simulink model "CubeSat_Archiv"  (R2019a)
settings: Solver=VariableStepAuto  StartTime=0.0  StopTime=10.0  RelTol=1e-3
undefined symbols (not defined in the file): D_distri, G_g, G_s, G_t, Gs, I_rw, I_vscmg, I_w, J_w, Kc, Ki, Kp, Kv, Kw_d, Kw_i, Kw_p, m, OMEGA_0, quat_0, smiData, tau_sat_mt, w_rw_ref, X, Y, Z
libraries: sm_lib x57, nesl_utility x28, aerolibutil x18, sharedtransform x5, ADCS_lib x4, simulink x2, sharedutil x2
(part 2 of 4)

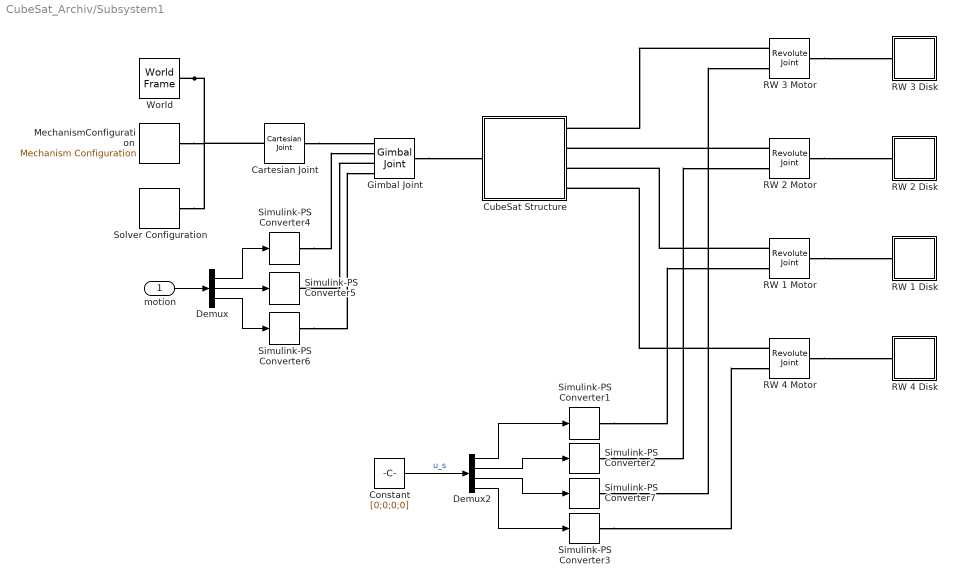
== system CubeSat_Archiv/Subsystem1 ==
  motion : Inport
  Cartesian Joint : sm_lib/Joints/Cartesian Joint  SenseConstraintForce=off  SenseConstraintForceX=off  SenseConstraintForceY=off  SenseConstraintForceZ=off  SenseConstraintTorque=off  SenseConstraintTorqueX=off  SenseConstraintTorqueY=off  SenseConstraintTorqueZ=off  SenseTotalForce=off  SenseTotalForceX=off  SenseTotalForceY=off  SenseTotalForceZ=off  SenseTotalTorque=off  SenseTotalTorqueX=off  SenseTotalTorqueY=off  SenseTotalTorqueZ=off  CompositeWrenchDir=FollowerOnBase  CompositeWrenchFrame=BaseFrame  PxEquilibriumPosition=0  PxEquilibriumPositionUnits=m  PxSpringStiffness=0  PxSpringStiffnessUnits=N/m  PxDampingCoefficient=0  PxDampingCoefficientUnits=N/(m/s)  PxTorqueActuationMode=NoTorque  PxMotionActuationMode=ComputedMotion  PxSensePosition=off  PxSenseVelocity=off  PxSenseAcceleration=off  PxSenseTorqueForce=off  PxSenseLowerLimitTorqueForce=off  PxSenseUpperLimitTorqueForce=off  PxLowerLimitSpecify=off  PxLowerLimitBound=-1  PxLowerLimitBoundUnits=m  PxLowerLimitStiffness=1e6  PxLowerLimitStiffnessUnits=N/m  PxLowerLimitDamping=1e3  PxLowerLimitDampingUnits=N/(m/s)  PxLowerLimitTransitionRegionWidth=1e-4  PxLowerLimitTransitionRegionWidthUnits=m  PxUpperLimitSpecify=off  PxUpperLimitBound=1  PxUpperLimitBoundUnits=m  PxUpperLimitStiffness=1e6  PxUpperLimitStiffnessUnits=N/m  PxUpperLimitDamping=1e3  PxUpperLimitDampingUnits=N/(m/s)  PxUpperLimitTransitionRegionWidth=1e-4  PxUpperLimitTransitionRegionWidthUnits=m  PxPositionTargetSpecify=off  PxPositionTargetPriority=High  PxPositionTargetValue=0  PxPositionTargetValueUnits=m  PxVelocityTargetSpecify=off  PxVelocityTargetPriority=High  PxVelocityTargetValue=0  PxVelocityTargetValueUnits=m/s  PyEquilibriumPosition=0  PyEquilibriumPositionUnits=m  PySpringStiffness=0  PySpringStiffnessUnits=N/m  PyDampingCoefficient=0  PyDampingCoefficientUnits=N/(m/s)  PyTorqueActuationMode=NoTorque  PyMotionActuationMode=ComputedMotion  PySensePosition=off  PySenseVelocity=off  PySenseAcceleration=off  PySenseTorqueForce=off  PySenseLowerLimitTorqueForce=off  PySenseUpperLimitTorqueForce=off  PyLowerLimitSpecify=off  PyLowerLimitBound=-1  PyLowerLimitBoundUnits=m  PyLowerLimitStiffness=1e6  PyLowerLimitStiffnessUnits=N/m  PyLowerLimitDamping=1e3  PyLowerLimitDampingUnits=N/(m/s)  PyLowerLimitTransitionRegionWidth=1e-4  PyLowerLimitTransitionRegionWidthUnits=m  PyUpperLimitSpecify=off  PyUpperLimitBound=1  PyUpperLimitBoundUnits=m  PyUpperLimitStiffness=1e6  PyUpperLimitStiffnessUnits=N/m  PyUpperLimitDamping=1e3  PyUpperLimitDampingUnits=N/(m/s)  PyUpperLimitTransitionRegionWidth=1e-4  PyUpperLimitTransitionRegionWidthUnits=m  PyPositionTargetSpecify=off  PyPositionTargetPriority=High  PyPositionTargetValue=0  PyPositionTargetValueUnits=m  PyVelocityTargetSpecify=off  PyVelocityTargetPriority=High  PyVelocityTargetValue=0  PyVelocityTargetValueUnits=m/s  PzEquilibriumPosition=0  PzEquilibriumPositionUnits=m  PzSpringStiffness=0  PzSpringStiffnessUnits=N/m  PzDampingCoefficient=0  PzDampingCoefficientUnits=N/(m/s)  PzTorqueActuationMode=NoTorque  PzMotionActuationMode=ComputedMotion  PzSensePosition=off  PzSenseVelocity=off  PzSenseAcceleration=off  PzSenseTorqueForce=off  PzSenseLowerLimitTorqueForce=off  PzSenseUpperLimitTorqueForce=off  PzLowerLimitSpecify=off  PzLowerLimitBound=-1  PzLowerLimitBoundUnits=m  PzLowerLimitStiffness=1e6  PzLowerLimitStiffnessUnits=N/m  PzLowerLimitDamping=1e3  PzLowerLimitDampingUnits=N/(m/s)  PzLowerLimitTransitionRegionWidth=1e-4  PzLowerLimitTransitionRegionWidthUnits=m  PzUpperLimitSpecify=off  PzUpperLimitBound=1  PzUpperLimitBoundUnits=m  PzUpperLimitStiffness=1e6  PzUpperLimitStiffnessUnits=N/m  PzUpperLimitDamping=1e3  PzUpperLimitDampingUnits=N/(m/s)  PzUpperLimitTransitionRegionWidth=1e-4  PzUpperLimitTransitionRegionWidthUnits=m  PzPositionTargetSpecify=off  PzPositionTargetPriority=High  PzPositionTargetValue=0  PzPositionTargetValueUnits=m  PzVelocityTargetSpecify=off  PzVelocityTargetPriority=High  PzVelocityTargetValue=0  PzVelocityTargetValueUnits=m/s
  Constant : Constant  Value=[0;0;0;0]
  CubeSat Structure : Subsystem
  Demux : Demux  Outputs=3
  Demux2 : Demux
  Gimbal Joint : sm_lib/Joints/Gimbal Joint  SenseConstraintForce=off  SenseConstraintForceX=off  SenseConstraintForceY=off  SenseConstraintForceZ=off  SenseConstraintTorque=off  SenseConstraintTorqueX=off  SenseConstraintTorqueY=off  SenseConstraintTorqueZ=off  SenseTotalForce=off  SenseTotalForceX=off  SenseTotalForceY=off  SenseTotalForceZ=off  SenseTotalTorque=off  SenseTotalTorqueX=off  SenseTotalTorqueY=off  SenseTotalTorqueZ=off  CompositeWrenchDir=FollowerOnBase  CompositeWrenchFrame=BaseFrame  RxEquilibriumPosition=0  RxEquilibriumPositionUnits=deg  RxSpringStiffness=0  RxSpringStiffnessUnits=N*m/deg  RxDampingCoefficient=0  RxDampingCoefficientUnits=N*m/(deg/s)  RxTorqueActuationMode=ComputedTorque  RxMotionActuationMode=InputMotion  RxSensePosition=off  RxSenseVelocity=off  RxSenseAcceleration=off  RxSenseTorqueForce=off  RxSenseLowerLimitTorqueForce=off  RxSenseUpperLimitTorqueForce=off  RxLowerLimitSpecify=off  RxLowerLimitBound=-90  RxLowerLimitBoundUnits=deg  RxLowerLimitStiffness=1e4  RxLowerLimitStiffnessUnits=N*m/deg  RxLowerLimitDamping=10  RxLowerLimitDampingUnits=N*m/(deg/s)  RxLowerLimitTransitionRegionWidth=0.1  RxLowerLimitTransitionRegionWidthUnits=deg  RxUpperLimitSpecify=off  RxUpperLimitBound=90  RxUpperLimitBoundUnits=deg  RxUpperLimitStiffness=1e4  RxUpperLimitStiffnessUnits=N*m/deg  RxUpperLimitDamping=10  RxUpperLimitDampingUnits=N*m/(deg/s)  RxUpperLimitTransitionRegionWidth=0.1  RxUpperLimitTransitionRegionWidthUnits=deg  RxPositionTargetSpecify=off  RxPositionTargetPriority=High  RxPositionTargetValue=0  RxPositionTargetValueUnits=rad  RxVelocityTargetSpecify=off  RxVelocityTargetPriority=High  RxVelocityTargetValue=0  RxVelocityTargetValueUnits=deg/s  RyEquilibriumPosition=0  RyEquilibriumPositionUnits=deg  RySpringStiffness=0  RySpringStiffnessUnits=N*m/deg  RyDampingCoefficient=0  RyDampingCoefficientUnits=N*m/(deg/s)  RyTorqueActuationMode=ComputedTorque  RyMotionActuationMode=InputMotion  RySensePosition=off  RySenseVelocity=off  RySenseAcceleration=off  RySenseTorqueForce=off  RySenseLowerLimitTorqueForce=off  RySenseUpperLimitTorqueForce=off  RyLowerLimitSpecify=off  RyLowerLimitBound=-90  RyLowerLimitBoundUnits=deg  RyLowerLimitStiffness=1e4  RyLowerLimitStiffnessUnits=N*m/deg  RyLowerLimitDamping=10  RyLowerLimitDampingUnits=N*m/(deg/s)  RyLowerLimitTransitionRegionWidth=0.1  RyLowerLimitTransitionRegionWidthUnits=deg  RyUpperLimitSpecify=off  RyUpperLimitBound=90  RyUpperLimitBoundUnits=deg  RyUpperLimitStiffness=1e4  RyUpperLimitStiffnessUnits=N*m/deg  RyUpperLimitDamping=10  RyUpperLimitDampingUnits=N*m/(deg/s)  RyUpperLimitTransitionRegionWidth=0.1  RyUpperLimitTransitionRegionWidthUnits=deg  RyPositionTargetSpecify=off  RyPositionTargetPriority=High  RyPositionTargetValue=0  RyPositionTargetValueUnits=deg  RyVelocityTargetSpecify=off  RyVelocityTargetPriority=High  RyVelocityTargetValue=0  RyVelocityTargetValueUnits=deg/s  RzEquilibriumPosition=0  RzEquilibriumPositionUnits=deg  RzSpringStiffness=0  RzSpringStiffnessUnits=N*m/deg  RzDampingCoefficient=0  RzDampingCoefficientUnits=N*m/(deg/s)  RzTorqueActuationMode=ComputedTorque  RzMotionActuationMode=InputMotion  RzSensePosition=off  RzSenseVelocity=off  RzSenseAcceleration=off  RzSenseTorqueForce=off  RzSenseLowerLimitTorqueForce=off  RzSenseUpperLimitTorqueForce=off  RzLowerLimitSpecify=off  RzLowerLimitBound=-90  RzLowerLimitBoundUnits=deg  RzLowerLimitStiffness=1e4  RzLowerLimitStiffnessUnits=N*m/deg  RzLowerLimitDamping=10  RzLowerLimitDampingUnits=N*m/(deg/s)  RzLowerLimitTransitionRegionWidth=0.1  RzLowerLimitTransitionRegionWidthUnits=deg  RzUpperLimitSpecify=off  RzUpperLimitBound=90  RzUpperLimitBoundUnits=deg  RzUpperLimitStiffness=1e4  RzUpperLimitStiffnessUnits=N*m/deg  RzUpperLimitDamping=10  RzUpperLimitDampingUnits=N*m/(deg/s)  RzUpperLimitTransitionRegionWidth=0.1  RzUpperLimitTransitionRegionWidthUnits=deg  RzPositionTargetSpecify=off  RzPositionTargetPriority=High  RzPositionTargetValue=0  RzPositionTargetValueUnits=deg  RzVelocityTargetSpecify=off  RzVelocityTargetPriority=High  RzVelocityTargetValue=0  RzVelocityTargetValueUnits=deg/s
      settings: SourceProductName=Simscape Multibody
  MechanismConfiguration : sm_lib/Utilities/Mechanism Configuration  UniformGravity=None  GravityVector=[0 -9.80665 0]  GravityUnits=m/s^2  LinearizationDelta=0.001
  RW 1 Disk : Subsystem
  RW 1 Motor : sm_lib/Joints/Revolute Joint  SenseConstraintForce=off  SenseConstraintForceX=off  SenseConstraintForceY=off  SenseConstraintForceZ=off  SenseConstraintTorque=off  SenseConstraintTorqueX=off  SenseConstraintTorqueY=off  SenseConstraintTorqueZ=off  SenseTotalForce=off  SenseTotalForceX=off  SenseTotalForceY=off  SenseTotalForceZ=off  SenseTotalTorque=off  SenseTotalTorqueX=off  SenseTotalTorqueY=off  SenseTotalTorqueZ=off  CompositeWrenchDir=FollowerOnBase  CompositeWrenchFrame=BaseFrame  EquilibriumPosition=0  EquilibriumPositionUnits=rad  SpringStiffness=0  SpringStiffnessUnits=N*m/rad  DampingCoefficient=0  DampingCoefficientUnits=N*m/(rad/s)  TorqueActuationMode=InputTorque  MotionActuationMode=ComputedMotion  SensePosition=off  SenseVelocity=off  SenseAcceleration=off  SenseTorqueForce=off  SenseLowerLimitTorqueForce=off  SenseUpperLimitTorqueForce=off  LowerLimitSpecify=off  LowerLimitBound=-90  LowerLimitBoundUnits=deg  LowerLimitStiffness=1e4  LowerLimitStiffnessUnits=N*m/deg  LowerLimitDamping=10  LowerLimitDampingUnits=N*m/(deg/s)  LowerLimitTransitionRegionWidth=0.1  LowerLimitTransitionRegionWidthUnits=deg  UpperLimitSpecify=off  UpperLimitBound=90  UpperLimitBoundUnits=deg  UpperLimitStiffness=1e4  UpperLimitStiffnessUnits=N*m/deg  UpperLimitDamping=10  UpperLimitDampingUnits=N*m/(deg/s)  UpperLimitTransitionRegionWidth=0.1  UpperLimitTransitionRegionWidthUnits=deg  PositionTargetSpecify=off  PositionTargetPriority=Low  PositionTargetValue=smiData.RevoluteJoint(2).Rz.Pos  PositionTargetValueUnits=deg  VelocityTargetSpecify=off  VelocityTargetPriority=High  VelocityTargetValue=0  VelocityTargetValueUnits=deg/s
  RW 2 Disk : Subsystem
  RW 2 Motor : sm_lib/Joints/Revolute Joint  SenseConstraintForce=off  SenseConstraintForceX=off  SenseConstraintForceY=off  SenseConstraintForceZ=off  SenseConstraintTorque=off  SenseConstraintTorqueX=off  SenseConstraintTorqueY=off  SenseConstraintTorqueZ=off  SenseTotalForce=off  SenseTotalForceX=off  SenseTotalForceY=off  SenseTotalForceZ=off  SenseTotalTorque=off  SenseTotalTorqueX=off  SenseTotalTorqueY=off  SenseTotalTorqueZ=off  CompositeWrenchDir=FollowerOnBase  CompositeWrenchFrame=BaseFrame  EquilibriumPosition=0  EquilibriumPositionUnits=rad  SpringStiffness=0  SpringStiffnessUnits=N*m/rad  DampingCoefficient=0  DampingCoefficientUnits=N*m/(rad/s)  TorqueActuationMode=InputTorque  MotionActuationMode=ComputedMotion  SensePosition=off  SenseVelocity=off  SenseAcceleration=off  SenseTorqueForce=off  SenseLowerLimitTorqueForce=off  SenseUpperLimitTorqueForce=off  LowerLimitSpecify=off  LowerLimitBound=-90  LowerLimitBoundUnits=deg  LowerLimitStiffness=1e4  LowerLimitStiffnessUnits=N*m/deg  LowerLimitDamping=10  LowerLimitDampingUnits=N*m/(deg/s)  LowerLimitTransitionRegionWidth=0.1  LowerLimitTransitionRegionWidthUnits=deg  UpperLimitSpecify=off  UpperLimitBound=90  UpperLimitBoundUnits=deg  UpperLimitStiffness=1e4  UpperLimitStiffnessUnits=N*m/deg  UpperLimitDamping=10  UpperLimitDampingUnits=N*m/(deg/s)  UpperLimitTransitionRegionWidth=0.1  UpperLimitTransitionRegionWidthUnits=deg  PositionTargetSpecify=off  PositionTargetPriority=Low  PositionTargetValue=smiData.RevoluteJoint(3).Rz.Pos  PositionTargetValueUnits=deg  VelocityTargetSpecify=off  VelocityTargetPriority=High  VelocityTargetValue=0  VelocityTargetValueUnits=deg/s
  RW 3 Disk : Subsystem
  RW 3 Motor : sm_lib/Joints/Revolute Joint  SenseConstraintForce=off  SenseConstraintForceX=off  SenseConstraintForceY=off  SenseConstraintForceZ=off  SenseConstraintTorque=off  SenseConstraintTorqueX=off  SenseConstraintTorqueY=off  SenseConstraintTorqueZ=off  SenseTotalForce=off  SenseTotalForceX=off  SenseTotalForceY=off  SenseTotalForceZ=off  SenseTotalTorque=off  SenseTotalTorqueX=off  SenseTotalTorqueY=off  SenseTotalTorqueZ=off  CompositeWrenchDir=FollowerOnBase  CompositeWrenchFrame=BaseFrame  EquilibriumPosition=0  EquilibriumPositionUnits=rad  SpringStiffness=0  SpringStiffnessUnits=N*m/rad  DampingCoefficient=0  DampingCoefficientUnits=N*m/(rad/s)  TorqueActuationMode=InputTorque  MotionActuationMode=ComputedMotion  SensePosition=off  SenseVelocity=off  SenseAcceleration=off  SenseTorqueForce=off  SenseLowerLimitTorqueForce=off  SenseUpperLimitTorqueForce=off  LowerLimitSpecify=off  LowerLimitBound=-90  LowerLimitBoundUnits=deg  LowerLimitStiffness=1e4  LowerLimitStiffnessUnits=N*m/deg  LowerLimitDamping=10  LowerLimitDampingUnits=N*m/(deg/s)  LowerLimitTransitionRegionWidth=0.1  LowerLimitTransitionRegionWidthUnits=deg  UpperLimitSpecify=off  UpperLimitBound=90  UpperLimitBoundUnits=deg  UpperLimitStiffness=1e4  UpperLimitStiffnessUnits=N*m/deg  UpperLimitDamping=10  UpperLimitDampingUnits=N*m/(deg/s)  UpperLimitTransitionRegionWidth=0.1  UpperLimitTransitionRegionWidthUnits=deg  PositionTargetSpecify=off  PositionTargetPriority=Low  PositionTargetValue=smiData.RevoluteJoint(4).Rz.Pos  PositionTargetValueUnits=deg  VelocityTargetSpecify=off  VelocityTargetPriority=High  VelocityTargetValue=0  VelocityTargetValueUnits=deg/s
  RW 4 Disk : Subsystem
  RW 4 Motor : sm_lib/Joints/Revolute Joint  SenseConstraintForce=off  SenseConstraintForceX=off  SenseConstraintForceY=off  SenseConstraintForceZ=off  SenseConstraintTorque=off  SenseConstraintTorqueX=off  SenseConstraintTorqueY=off  SenseConstraintTorqueZ=off  SenseTotalForce=off  SenseTotalForceX=off  SenseTotalForceY=off  SenseTotalForceZ=off  SenseTotalTorque=off  SenseTotalTorqueX=off  SenseTotalTorqueY=off  SenseTotalTorqueZ=off  CompositeWrenchDir=FollowerOnBase  CompositeWrenchFrame=BaseFrame  EquilibriumPosition=0  EquilibriumPositionUnits=rad  SpringStiffness=0  SpringStiffnessUnits=N*m/rad  DampingCoefficient=0  DampingCoefficientUnits=N*m/(rad/s)  TorqueActuationMode=InputTorque  MotionActuationMode=ComputedMotion  SensePosition=off  SenseVelocity=off  SenseAcceleration=off  SenseTorqueForce=off  SenseLowerLimitTorqueForce=off  SenseUpperLimitTorqueForce=off  LowerLimitSpecify=off  LowerLimitBound=-90  LowerLimitBoundUnits=deg  LowerLimitStiffness=1e4  LowerLimitStiffnessUnits=N*m/deg  LowerLimitDamping=10  LowerLimitDampingUnits=N*m/(deg/s)  LowerLimitTransitionRegionWidth=0.1  LowerLimitTransitionRegionWidthUnits=deg  UpperLimitSpecify=off  UpperLimitBound=90  UpperLimitBoundUnits=deg  UpperLimitStiffness=1e4  UpperLimitStiffnessUnits=N*m/deg  UpperLimitDamping=10  UpperLimitDampingUnits=N*m/(deg/s)  UpperLimitTransitionRegionWidth=0.1  UpperLimitTransitionRegionWidthUnits=deg  PositionTargetSpecify=off  PositionTargetPriority=Low  PositionTargetValue=smiData.RevoluteJoint(1).Rz.Pos  PositionTargetValueUnits=deg  VelocityTargetSpecify=off  VelocityTargetPriority=High  VelocityTargetValue=0  VelocityTargetValueUnits=deg/s
  Simulink-PS Converter{1,4..6} (4 alike) : nesl_utility/Simulink-PS Converter  PhysicalDomain=network_engine_domain  SubClassName=ps_input  LeftPortType=input  RightPortType=output  PseudoPeriodic=off  Frequencies=[]  NoiseDistribution=none  NoiseParameters=[]  Unit=1  AffineConversion=off  FilteringAndDerivatives=filter  SimscapeFilterOrder=2  InputFilterTimeConstant=0.001  UdotUserProvided=1
  Simulink-PS Converter2 : nesl_utility/Simulink-PS Converter  PhysicalDomain=network_engine_domain  SubClassName=ps_input  LeftPortType=input  RightPortType=output  PseudoPeriodic=off  Frequencies=[]  NoiseDistribution=none  NoiseParameters=[]  Unit=1  AffineConversion=off  FilteringAndDerivatives=filter  SimscapeFilterOrder=2  InputFilterTimeConstant=0.001  UdotUserProvided=0
  Simulink-PS Converter3 : nesl_utility/Simulink-PS Converter  PhysicalDomain=network_engine_domain  SubClassName=ps_input  LeftPortType=input  RightPortType=output  PseudoPeriodic=off  Frequencies=[]  NoiseDistribution=none  NoiseParameters=[]  Unit=1  AffineConversion=off  FilteringAndDerivatives=filter  SimscapeFilterOrder=2  InputFilterTimeConstant=0.001  UdotUserProvided=0
  Simulink-PS Converter7 : nesl_utility/Simulink-PS Converter  PhysicalDomain=network_engine_domain  SubClassName=ps_input  LeftPortType=input  RightPortType=output  PseudoPeriodic=off  Frequencies=[]  NoiseDistribution=none  NoiseParameters=[]  Unit=1  AffineConversion=off  FilteringAndDerivatives=filter  SimscapeFilterOrder=2  InputFilterTimeConstant=0.001  UdotUserProvided=0
  Solver Configuration : nesl_utility/Solver Configuration  PhysicalDomain=network_engine_domain  SubClassName=solver  LeftPortType=input  RightPortType=generic  Tones=[]  Harmonics=[]  SimulateNoise=off  Profile=off  UseLocalSampling=off  EnableSwitchedLinearOptims=on  FrequencyDomain=off  UseCCode=off  RelTol=0.001  AbsTol=1e-06  MinStep=1e-09  ToWorkspace=off  RevertToSquareIcSolve=off  NumHomotopyIterations=100  PhasorMode=off  PhasorModeNumHarmonics=1  DoDC=off  ResidualTolerance=1e-09  UseLocalSolver=off  LocalSolverChoice=NE_BACKWARD_EULER_ADVANCER  LocalSolverSampleTime=0.001  DoFixedCost=off  MaxNonlinIter=3  MaxModeIter=2  LinearAlgebra=Sparse  EquationFormulation=NE_TIME_EF  DelaysMemoryBudget=1024  AutomaticFiltering=on  FilteringTimeConstant=0.001  PartitionStorageMethod=AS_NEEDED  PartitionMemoryBudget=1024  PartitionMethod=FAST
  World : sm_lib/Frames and Transforms/World Frame
  wires:
  Demux2/2 -> Simulink-PS Converter2/1
  Demux2/3 -> Simulink-PS Converter7/1
  Demux2/4 -> Simulink-PS Converter3/1
  Demux2/1 -> Simulink-PS Converter1/1
  Constant/1 -> Demux2/1  "u_s"
  Demux/2 -> Simulink-PS Converter5/1
  Demux/1 -> Simulink-PS Converter4/1
  Demux/3 -> Simulink-PS Converter6/1
  motion/1 -> Demux/1
  connections:
  World/RConn1 -- Cartesian Joint/LConn1 -- Solver Configuration/RConn1 -- MechanismConfiguration/RConn1
  Simulink-PS Converter3/RConn1 -- RW 4 Motor/LConn2
  RW 3 Motor/RConn1 -- RW 3 Disk/LConn1
  Simulink-PS Converter1/RConn1 -- RW 1 Motor/LConn2
  Simulink-PS Converter7/RConn1 -- RW 3 Motor/LConn2
  RW 2 Motor/RConn1 -- RW 2 Disk/LConn1
  Simulink-PS Converter2/RConn1 -- RW 2 Motor/LConn2
  RW 1 Motor/RConn1 -- RW 1 Disk/LConn1
  RW 4 Motor/LConn1 -- CubeSat Structure/RConn4
  RW 1 Motor/LConn1 -- CubeSat Structure/RConn3
  RW 3 Motor/LConn1 -- CubeSat Structure/RConn1
  RW 4 Motor/RConn1 -- RW 4 Disk/LConn1
  RW 2 Motor/LConn1 -- CubeSat Structure/RConn2
  Gimbal Joint/RConn1 -- CubeSat Structure/LConn1
  Cartesian Joint/RConn1 -- Gimbal Joint/LConn1
  Simulink-PS Converter4/RConn1 -- Gimbal Joint/LConn2
  Gimbal Joint/LConn3 -- Simulink-PS Converter5/RConn1
  Simulink-PS Converter6/RConn1 -- Gimbal Joint/LConn4

== system CubeSat_Archiv/vscmg dynamics v1.0 ==
  note: VSCMG Eqn
  In1 : Inport
  In2 : Inport  Port=2
  Dynamics VSCMG : Subsystem
  Kinematics1 : Subsystem
  OMEGA_vscmg : Scope
  VSCMGC : Subsystem
  omega_w_vscmg : Scope
  Out1 : Outport
  wires:
  Kinematics1/1(q) -> Out1/1
  In2/1 -> Dynamics VSCMG/3(ext.torq)
  Dynamics VSCMG/1(OMEGA) -> OMEGA_vscmg/1, Kinematics1/1(OMEGA)
  Dynamics VSCMG/2(ALPHA) -> VSCMGC/1(ALPHA)
  VSCMGC/2(alpha_w) -> Dynamics VSCMG/2(alpha_w)
  In1/1 -> VSCMGC/2(tau_cmd)
  VSCMGC/1(omega_w) -> Dynamics VSCMG/1(omega_w), omega_w_vscmg/1

== system CubeSat_Archiv/Actuator/Magnetic Torquer Cluster ==
  b_t_cmd_mtc : Inport
  Envi : Inport  Port=2
  Terminator : Terminator
  Out1 : Outport
  wires:
  b_t_cmd_mtc/1 -> Out1/1
  Envi/1 -> Terminator/1

== system CubeSat_Archiv/Actuator/Reaction Wheel Cluster ==
  b_w_b/n : Inport
  b_a_b/n : Inport  Port=2
  b_t_cmd_rwc : Inport  Port=3
  Demux : Demux
  Distri Mtx2 : Gain  Gain=D_distri  Multiplication=Matrix(K*u)
  Mux1 : Mux
  Mux2 : Mux
  RW 1 : Subsystem
  RW 2 : Subsystem
  RW 3 : Subsystem
  RW 4 : Subsystem
  h_s : Outport
  u_s : Outport  Port=2
  omega_w : Outport  Port=3
  wires:
  Demux/3 -> RW 3/3(u_s_3)
  Demux/1 -> RW 1/3(u_s_1)
  Demux/2 -> RW 2/3(u_s_2)
  Demux/4 -> RW 4/3(u_s_4)
  b_t_cmd_rwc/1 -> Distri Mtx2/1
  b_a_b/n/1 -> RW 4/2(ALPHA), RW 3/2(ALPHA), RW 2/2(ALPHA), RW 1/2(ALPHA)
  RW 1/2(omega_w_1) -> Mux2/1
  Distri Mtx2/1 -> u_s/1, Demux/1  "u_s"
  RW 4/1(h_w_4) -> Mux1/4
  RW 1/1(h_w_1) -> Mux1/1
  Mux2/1 -> omega_w/1
  Mux1/1 -> h_s/1
  RW 3/2(omega_w_3) -> Mux2/3
  RW 4/2(omega_w_4) -> Mux2/4
  b_w_b/n/1 -> RW 4/1(OMEGA), RW 3/1(OMEGA), RW 2/1(OMEGA), RW 1/1(OMEGA)
  RW 3/1(h_w_3) -> Mux1/3
  RW 2/2(omega_w_2) -> Mux2/2
  RW 2/1(h_w_2) -> Mux1/2

== system CubeSat_Archiv/Controller1/LQI_Full State_Verified1 ==
  In Bus Element2 : Inport  PortName=RefState  Element=q_eci2r
  In Bus Element : Inport  Port=2  PortName=SensorIn  Element=q_eci2b
  In Bus Element7 : Inport  Port=2  PortName=SensorIn  Element=b_w_b/n
  Add2 : Sum  Inputs=|+-
  Atti Err : Subsystem  AncestorBlock=ADCS_lib/PIV/Atti Err
  Integrator1 : Integrator
  Kc Ctrl Gain : Gain  Gain=-Kc  Multiplication=Matrix(K*u)
  Ki Integral Gain : Gain  Gain=Ki  Multiplication=Matrix(K*u)
  Vector Concatenate : Concatenate
  Vector Concatenate1 : Concatenate
  Vector Out Unwinding1 : Subsystem
  vector part1 : Selector  InputPortWidth=4  IndexOptions=Index vector (dialog)  Indices=[2 3 4]  OutputSizes=1
  CtrlCmd : Outport
  Out Bus Element : Outport  Port=2  PortName=CtrlState  Element=q_r2b
  wires:
  Ki Integral Gain/1 -> Add2/1
  Atti Err/1(q_r2b) -> Out Bus Element/1, Vector Out Unwinding1/1(q)
  In Bus Element/1 -> vector part1/1, Atti Err/2(q_eci2b)
  In Bus Element2/1 -> Atti Err/1(q_eci2r)
  Kc Ctrl Gain/1 -> Add2/2
  Add2/1 -> CtrlCmd/1
  Integrator1/1 -> Ki Integral Gain/1
  vector part1/1 -> Vector Concatenate/1
  Vector Concatenate/1 -> Kc Ctrl Gain/1
  In Bus Element7/1 -> Vector Concatenate/2, Vector Concatenate1/2
  Vector Out Unwinding1/1(ε) -> Vector Concatenate1/1
  Vector Concatenate1/1 -> Integrator1/1

== system CubeSat_Archiv/Controller1/Momentum Management ==
  CtrlCmd : Inport
  w_rw : Inport  Port=2
  Add : Sum  Inputs=|++
  G_s : Gain  Gain=G_s  Multiplication=Matrix(K*u)
  de-spin torq : Subsystem
  b_t_cmd_rwc : Outport
  b_t_cmd_mtc : Outport  Port=2
  wires:
  de-spin torq/1(u_despin) -> G_s/1
  w_rw/1 -> de-spin torq/1(w_rw)
  Add/1 -> b_t_cmd_rwc/1
  G_s/1 -> b_t_cmd_mtc/1, Add/2
  CtrlCmd/1 -> Add/1

== system CubeSat_Archiv/Dynamics/integrate quaternion ==
  b_w_b/n : Inport
  Constant : Constant  Value=0
  Gain : Gain  Gain=0.5
  Integrator : Integrator  InitialCondition=quat_0
  Quaternion Multiplication : aerolibutil/Quaternion Multiplication
  Vector Concatenate : Concatenate
  q_eci2b : Outport
  wires:
  Quaternion Multiplication/1 -> Integrator/1
  b_w_b/n/1 -> Vector Concatenate/2
  Integrator/1 -> q_eci2b/1, Gain/1
  Gain/1 -> Quaternion Multiplication/1
  Vector Concatenate/1 -> Quaternion Multiplication/2
  Constant/1 -> Vector Concatenate/1

== system CubeSat_Archiv/Dynamics without FF/Integrate Quaternion KDE ==
  b_w_b/n : Inport
  Constant : Constant  Value=0
  Gain : Gain  Gain=0.5
  Integrator : Integrator  InitialCondition=quat_0
  Quaternion Multiplication : aerolibutil/Quaternion Multiplication
  Quaternion Normalize : sharedutil/Quaternion Normalize  aMode=aMode
      settings: SourceProductName=Aerospace Blockset  SourceProductBaseCode=AE
  Vector Concatenate : Concatenate
  q_eci2b : Outport
  wires:
  Quaternion Normalize/1 -> q_eci2b/1
  Constant/1 -> Vector Concatenate/1
  Vector Concatenate/1 -> Quaternion Multiplication/2
  Gain/1 -> Quaternion Multiplication/1
  Integrator/1 -> Gain/1, Quaternion Normalize/1
  b_w_b/n/1 -> Vector Concatenate/2
  Quaternion Multiplication/1 -> Integrator/1

== system CubeSat_Archiv/FeedFwd/RW 1 ==
  OMEGA : Inport
  omega_w_1 : Inport  Port=2
  Gain2 : Gain  Gain=G_s(:,1).'  Multiplication=Matrix(K*u)
  I_w : Gain  Gain=I_w(1,1)
  Sum1 : Sum
  h_w_1 : Outport
  wires:
  omega_w_1/1 -> Sum1/2
  Sum1/1 -> I_w/1
  I_w/1 -> h_w_1/1
  Gain2/1 -> Sum1/1
  OMEGA/1 -> Gain2/1

== system CubeSat_Archiv/FeedFwd/RW 2 ==
  OMEGA : Inport
  omega_w_1 : Inport  Port=2
  Gain2 : Gain  Gain=G_s(:,1).'  Multiplication=Matrix(K*u)
  I_w : Gain  Gain=I_w(1,1)
  Sum1 : Sum
  h_w_1 : Outport
  wires:
  OMEGA/1 -> Gain2/1
  Gain2/1 -> Sum1/1
  I_w/1 -> h_w_1/1
  Sum1/1 -> I_w/1
  omega_w_1/1 -> Sum1/2

== system CubeSat_Archiv/FeedFwd/RW 3 ==
  OMEGA : Inport
  omega_w_1 : Inport  Port=2
  Gain2 : Gain  Gain=G_s(:,1).'  Multiplication=Matrix(K*u)
  I_w : Gain  Gain=I_w(1,1)
  Sum1 : Sum
  h_w_1 : Outport
  wires:
  omega_w_1/1 -> Sum1/2
  Sum1/1 -> I_w/1
  I_w/1 -> h_w_1/1
  Gain2/1 -> Sum1/1
  OMEGA/1 -> Gain2/1

== system CubeSat_Archiv/FeedFwd/RW 4 ==
  OMEGA : Inport
  omega_w_1 : Inport  Port=2
  Gain2 : Gain  Gain=G_s(:,1).'  Multiplication=Matrix(K*u)
  I_w : Gain  Gain=I_w(1,1)
  Sum1 : Sum
  h_w_1 : Outport
  wires:
  OMEGA/1 -> Gain2/1
  Gain2/1 -> Sum1/1
  I_w/1 -> h_w_1/1
  Sum1/1 -> I_w/1
  omega_w_1/1 -> Sum1/2

== system CubeSat_Archiv/LQI_Full State_Verified/Atti Err1 ==
  q_eci2r : Inport
  q_eci2b : Inport  Port=2
  Quaternion Inverse1 : aerolibutil/Quaternion Inverse
      settings: SourceProductName=Aerospace Blockset
  Quaternion Multiplication : aerolibutil/Quaternion Multiplication
  "[BR]" : sharedtransform/Quaternions to  Direction Cosine Matrix  aMode=aMode
      settings: SourceProductName=Aerospace Blockset  SourceProductBaseCode=AE
  q_r2b : Outport
  DCM : Outport  Port=2
  wires:
  Quaternion Inverse1/1 -> Quaternion Multiplication/1
  "[BR]"/1 -> DCM/1
  q_eci2r/1 -> Quaternion Multiplication/2
  q_eci2b/1 -> Quaternion Inverse1/1
  Quaternion Multiplication/1 -> "[BR]"/1, q_r2b/1

== system CubeSat_Archiv/LQI_Full State_Verified/Vector Out Unwinding1 ==
  q : Inport
  Product2 : Product
  Short Rotation : Subsystem
  vector part : Selector  InputPortWidth=4  IndexOptions=Index vector (dialog)  Indices=[2 3 4]  OutputSizes=1
  ε : Outport
  wires:
  Product2/1 -> ε/1
  Short Rotation/1(sgn) -> Product2/1
  q/1 -> Short Rotation/1(q), vector part/1
  vector part/1 -> Product2/2

== system CubeSat_Archiv/LQI_Full State_Verified/r2b ==
  "[BR]" : Inport
  r_w_r/n : Inport  Port=2
  Derivative : Derivative
  Product : Product  Multiplication=Matrix(*)
  Product1 : Product  Multiplication=Matrix(*)
  b_w_r/n : Outport
  b_a_r/n : Outport  Port=2
  wires:
  Product/1 -> b_w_r/n/1
  Product1/1 -> b_a_r/n/1
  Derivative/1 -> Product1/2  "r_a_r/n"
  "[BR]"/1 -> Product/1, Product1/1
  r_w_r/n/1 -> Derivative/1, Product/2

== system CubeSat_Archiv/LQI_Half State_Don't Use!/Atti Err1 ==
  q_eci2r : Inport
  q_eci2b : Inport  Port=2
  Quaternion Inverse1 : aerolibutil/Quaternion Inverse
      settings: SourceProductName=Aerospace Blockset
  Quaternion Multiplication : aerolibutil/Quaternion Multiplication
  q_r2b : Outport
  wires:
  Quaternion Multiplication/1 -> q_r2b/1
  q_eci2b/1 -> Quaternion Inverse1/1
  q_eci2r/1 -> Quaternion Multiplication/2
  Quaternion Inverse1/1 -> Quaternion Multiplication/1

== system CubeSat_Archiv/LQI_Half State_Don't Use!/Vector Out Unwinding2 ==
  q : Inport
  Product2 : Product
  Short Rotation : Subsystem
  vector part : Selector  InputPortWidth=4  IndexOptions=Index vector (dialog)  Indices=[2 3 4]  OutputSizes=1
  ε : Outport
  wires:
  vector part/1 -> Product2/2
  q/1 -> vector part/1, Short Rotation/1(q)
  Short Rotation/1(sgn) -> Product2/1
  Product2/1 -> ε/1

== system CubeSat_Archiv/LQR Compensated_Verified/Atti Err ==
  q_eci2r : Inport
  q_eci2b : Inport  Port=2
  Quaternion Inverse1 : aerolibutil/Quaternion Inverse
      settings: SourceProductName=Aerospace Blockset
  Quaternion Multiplication : aerolibutil/Quaternion Multiplication
  "[BR]" : sharedtransform/Quaternions to  Direction Cosine Matrix  aMode=aMode
      settings: SourceProductName=Aerospace Blockset  SourceProductBaseCode=AE
  q_r2b : Outport
  DCM : Outport  Port=2
  wires:
  Quaternion Inverse1/1 -> Quaternion Multiplication/1
  "[BR]"/1 -> DCM/1
  q_eci2r/1 -> Quaternion Multiplication/2
  q_eci2b/1 -> Quaternion Inverse1/1
  Quaternion Multiplication/1 -> "[BR]"/1, q_r2b/1

== system CubeSat_Archiv/LQR Compensated_Verified/Vector Out Unwinding ==
  q : Inport
  Product2 : Product
  Short Rotation : Subsystem
  vector part : Selector  InputPortWidth=4  IndexOptions=Index vector (dialog)  Indices=[2 3 4]  OutputSizes=1
  ε : Outport
  wires:
  vector part/1 -> Product2/2
  q/1 -> vector part/1, Short Rotation/1(q)
  Short Rotation/1(sgn) -> Product2/1
  Product2/1 -> ε/1

== system CubeSat_Archiv/LQR Compensated_Verified/r2b ==
  "[BR]" : Inport
  r_w_r/n : Inport  Port=2
  Derivative : Derivative
  Product : Product  Multiplication=Matrix(*)
  Product1 : Product  Multiplication=Matrix(*)
  b_w_r/n : Outport
  b_a_r/n : Outport  Port=2
  wires:
  Product/1 -> b_w_r/n/1
  Product1/1 -> b_a_r/n/1
  Derivative/1 -> Product1/2  "r_a_r/n"
  "[BR]"/1 -> Product/1, Product1/1
  r_w_r/n/1 -> Derivative/1, Product/2

== system CubeSat_Archiv/Momentum Management1/de-spin torq ==
  w_rw : Inport
  Add : Sum  Inputs=+-
  Gain : Gain  Gain=-1
  I_w : Gain  Gain=I_w(1,:).'
  PID Controller1 : simulink/Continuous/PID Controller  Controller=PID  Form=Parallel  TimeDomain=Continuous-time  SampleTime=-1  IntegratorMethod=Forward Euler  FilterMethod=Forward Euler  ControllerParametersSource=internal  P=Kw_p  I=Kw_i  D=Kw_d  UseFilter=on  N=10  TunerSelectOption=Transfer Function Based (PID Tuner App)  InitialConditionSource=internal  InitialConditionForIntegrator=0  InitialConditionForFilter=0  DifferentiatorICPrevScaledInput=0  ExternalReset=none  TrackingMode=off  Kt=1  LimitOutput=off  UpperSaturationLimit=tau_sat_mt  LowerSaturationLimit=-tau_sat_mt  LinearizeAsGain=on  AntiWindupMode=clamping  Kb=1  POutMin=[]  POutMax=[]  IOutMin=[]  IOutMax=[]  DOutMin=[]  DOutMax=[]  NOutMin=[]  NOutMax=[]  SumOutMin=[]  SumOutMax=[]  SaturationOutMin=[]  SaturationOutMax=[]  PParamMin=[]  PParamMax=[]  IParamMin=[]  IParamMax=[]  DParamMin=[]  DParamMax=[]  NParamMin=[]  NParamMax=[]  KbParamMin=[]  KbParamMax=[]  KtParamMin=[]  KtParamMax=[]  KbOutMin=[]  KbOutMax=[]  KtOutMin=[]  KtOutMax=[]  IntegratorOutMin=[]  IntegratorOutMax=[]  FilterOutMin=[]  FilterOutMax=[]  SumI1OutMin=[]  SumI1OutMax=[]  SumI2OutMin=[]  SumI2OutMax=[]  SumI3OutMin=[]  SumI3OutMax=[]  SumI4OutMin=[]  SumI4OutMax=[]  SumDOutMin=[]  SumDOutMax=[]  DifferentiatorOutMin=[]  DifferentiatorOutMax=[]  FilterDiffOutCoefMin=[]  FilterDiffOutCoefMax=[]  ReciprocalOutMin=[]  ReciprocalOutMax=[]  SumDenOutMin=[]  SumDenOutMax=[]  SumNumOutMin=[]  SumNumOutMax=[]  DivideOutMin=[]  DivideOutMax=[]  IntegratorContinuousStateAttributes=''  IntegratorStateMustResolveToSignalObject=off  IntegratorRTWStateStorageClass=Auto  FilterContinuousStateAttributes=''  FilterStateMustResolveToSignalObject=off  FilterRTWStateStorageClass=Auto  ParallelPVariant=InternalParameters  IdealPVariant=Disabled  IVariant=InternalParameters  DVariant=InternalParameters  IntegratorVariant=Continuous  SatVariant=Disabled  AWVariant=Passthrough  PCopyVariant=Disabled  TRVariant=Disabled  FdbkBlocksVariant=Forward  IdealPFdbkVariant=Disabled  SatFdbkVariant=Disabled  DerivativeFilterVariant=ContFilter  NVariant=InternalParameters  NCopyVariant=Disabled  FilterICVariant=InternalICsFilter  IntegratorICVariant=InternalICs  ExternalResetVariant=Disabled  TRSumVariant=Passthrough  SumFdbkVariant=Disabled  SumVariant=Sum_PID
  w_rw_ref : Constant  Value=w_rw_ref
  u_despin : Outport
  wires:
  I_w/1 -> PID Controller1/1
  w_rw_ref/1 -> Add/2
  PID Controller1/1 -> Gain/1
  Gain/1 -> u_despin/1
  Add/1 -> I_w/1
  w_rw/1 -> Add/1

== system CubeSat_Archiv/PIV Compact No Feedfwd_Verified/Atti Err ==
  q_eci2r : Inport
  q_eci2b : Inport  Port=2
  Quaternion Inverse1 : aerolibutil/Quaternion Inverse
      settings: SourceProductName=Aerospace Blockset
  Quaternion Multiplication : aerolibutil/Quaternion Multiplication
  "[BR]" : sharedtransform/Quaternions to  Direction Cosine Matrix  aMode=aMode
      settings: SourceProductName=Aerospace Blockset  SourceProductBaseCode=AE
  q_r2b : Outport
  DCM_[BR] : Outport  Port=2
  wires:
  Quaternion Inverse1/1 -> Quaternion Multiplication/1
  "[BR]"/1 -> DCM_[BR]/1
  q_eci2r/1 -> Quaternion Multiplication/2
  q_eci2b/1 -> Quaternion Inverse1/1
  Quaternion Multiplication/1 -> "[BR]"/1, q_r2b/1

== system CubeSat_Archiv/PIV Compact No Feedfwd_Verified/Vector Out Unwinding ==
  q : Inport
  Product2 : Product
  Short Rotation : Subsystem
  vector part : Selector  InputPortWidth=4  IndexOptions=Index vector (dialog)  Indices=[2 3 4]  OutputSizes=1
  ε : Outport
  wires:
  vector part/1 -> Product2/2
  q/1 -> vector part/1, Short Rotation/1(q)
  Short Rotation/1(sgn) -> Product2/1
  Product2/1 -> ε/1

== system CubeSat_Archiv/PIV Compact No Feedfwd_Verified/Vector Out Unwinding1 ==
  q : Inport
  Product2 : Product
  Short Rotation : Subsystem
  vector part : Selector  InputPortWidth=4  IndexOptions=Index vector (dialog)  Indices=[2 3 4]  OutputSizes=1
  ε : Outport
  wires:
  Product2/1 -> ε/1
  Short Rotation/1(sgn) -> Product2/1
  q/1 -> Short Rotation/1(q), vector part/1
  vector part/1 -> Product2/2

== system CubeSat_Archiv/PIV Compact No Feedfwd_Verified/r2b ==
  "[BR]" : Inport
  r_w_r/n : Inport  Port=2
  Derivative : Derivative
  Product : Product  Multiplication=Matrix(*)
  Product1 : Product  Multiplication=Matrix(*)
  b_w_r/n : Outport
  b_a_r/n : Outport  Port=2
  wires:
  Product/1 -> b_w_r/n/1
  Product1/1 -> b_a_r/n/1
  Derivative/1 -> Product1/2  "r_a_r/n"
  "[BR]"/1 -> Product/1, Product1/1
  r_w_r/n/1 -> Derivative/1, Product/2

== system CubeSat_Archiv/PIV Full EoM_Verified/Atti Err ==
  q_eci2r : Inport
  q_eci2b : Inport  Port=2
  Quaternion Inverse1 : aerolibutil/Quaternion Inverse
      settings: SourceProductName=Aerospace Blockset
  Quaternion Multiplication : aerolibutil/Quaternion Multiplication
  "[BR]" : sharedtransform/Quaternions to  Direction Cosine Matrix  aMode=aMode
      settings: SourceProductName=Aerospace Blockset  SourceProductBaseCode=AE
  q_r2b : Outport
  DCM_[BR] : Outport  Port=2
  wires:
  Quaternion Inverse1/1 -> Quaternion Multiplication/1
  "[BR]"/1 -> DCM_[BR]/1
  q_eci2r/1 -> Quaternion Multiplication/2
  q_eci2b/1 -> Quaternion Inverse1/1
  Quaternion Multiplication/1 -> "[BR]"/1, q_r2b/1

== system CubeSat_Archiv/PIV Full EoM_Verified/Rate Err1 ==
  b_w_r/n : Inport
  b_w_b/n : Inport  Port=2
  Add1 : Sum  Inputs=+-
  b_deltaw_b/r : Outport
  wires:
  Add1/1 -> b_deltaw_b/r/1
  b_w_b/n/1 -> Add1/1
  b_w_r/n/1 -> Add1/2

== system CubeSat_Archiv/PIV Full EoM_Verified/Short Rotation1 ==
  q : Inport
  Gain1 : Gain  Gain=-1
  Sign1 : Signum
  extract scalar part : Selector  InputPortWidth=4  IndexOptions=Index vector (dialog)  Indices=[1]  OutputSizes=1
  sgn : Outport
  wires:
  Gain1/1 -> sgn/1
  Sign1/1 -> Gain1/1
  extract scalar part/1 -> Sign1/1
  q/1 -> extract scalar part/1

== system CubeSat_Archiv/PIV Full EoM_Verified/Short Rotation2 ==
  q : Inport
  Gain1 : Gain  Gain=-1
  Sign1 : Signum
  extract scalar part : Selector  InputPortWidth=4  IndexOptions=Index vector (dialog)  Indices=[1]  OutputSizes=1
  sgn : Outport
  wires:
  q/1 -> extract scalar part/1
  extract scalar part/1 -> Sign1/1
  Sign1/1 -> Gain1/1
  Gain1/1 -> sgn/1

== system CubeSat_Archiv/PIV Full EoM_Verified/r2b ==
  "[BR]" : Inport
  r_w_r/n : Inport  Port=2
  Derivative : Derivative
  Product : Product  Multiplication=Matrix(*)
  Product1 : Product  Multiplication=Matrix(*)
  b_w_r/n : Outport
  b_a_r/n : Outport  Port=2
  wires:
  Product/1 -> b_w_r/n/1
  Product1/1 -> b_a_r/n/1
  Derivative/1 -> Product1/2  "r_a_r/n"
  "[BR]"/1 -> Product/1, Product1/1
  r_w_r/n/1 -> Derivative/1, Product/2

== system CubeSat_Archiv/PIV No Feedfwd_Verified/Atti Err ==
  q_eci2r : Inport
  q_eci2b : Inport  Port=2
  Quaternion Inverse1 : aerolibutil/Quaternion Inverse
      settings: SourceProductName=Aerospace Blockset
  Quaternion Multiplication : aerolibutil/Quaternion Multiplication
  "[BR]" : sharedtransform/Quaternions to  Direction Cosine Matrix  aMode=aMode
      settings: SourceProductName=Aerospace Blockset  SourceProductBaseCode=AE
  q_r2b : Outport
  DCM_[BR] : Outport  Port=2
  wires:
  Quaternion Multiplication/1 -> q_r2b/1, "[BR]"/1
  q_eci2b/1 -> Quaternion Inverse1/1
  q_eci2r/1 -> Quaternion Multiplication/2
  "[BR]"/1 -> DCM_[BR]/1
  Quaternion Inverse1/1 -> Quaternion Multiplication/1

== system CubeSat_Archiv/PIV No Feedfwd_Verified/Rate Err1 ==
  b_w_r/n : Inport
  b_w_b/n : Inport  Port=2
  Add1 : Sum  Inputs=+-
  b_deltaw_b/r : Outport
  wires:
  b_w_r/n/1 -> Add1/2
  b_w_b/n/1 -> Add1/1
  Add1/1 -> b_deltaw_b/r/1

== system CubeSat_Archiv/PIV No Feedfwd_Verified/Short Rotation1 ==
  q : Inport
  Gain1 : Gain  Gain=-1
  Sign1 : Signum
  extract scalar part : Selector  InputPortWidth=4  IndexOptions=Index vector (dialog)  Indices=[1]  OutputSizes=1
  sgn : Outport
  wires:
  q/1 -> extract scalar part/1
  extract scalar part/1 -> Sign1/1
  Sign1/1 -> Gain1/1
  Gain1/1 -> sgn/1

== system CubeSat_Archiv/PIV No Feedfwd_Verified/Short Rotation2 ==
  q : Inport
  Gain1 : Gain  Gain=-1
  Sign1 : Signum
  extract scalar part : Selector  InputPortWidth=4  IndexOptions=Index vector (dialog)  Indices=[1]  OutputSizes=1
  sgn : Outport
  wires:
  Gain1/1 -> sgn/1
  Sign1/1 -> Gain1/1
  extract scalar part/1 -> Sign1/1
  q/1 -> extract scalar part/1

== system CubeSat_Archiv/PIV No Feedfwd_Verified/r2b ==
  "[BR]" : Inport
  r_w_r/n : Inport  Port=2
  Derivative : Derivative
  Product : Product  Multiplication=Matrix(*)
  Product1 : Product  Multiplication=Matrix(*)
  b_w_r/n : Outport
  b_a_r/n : Outport  Port=2
  wires:
  r_w_r/n/1 -> Product/2, Derivative/1
  "[BR]"/1 -> Product1/1, Product/1
  Derivative/1 -> Product1/2  "r_a_r/n"
  Product1/1 -> b_a_r/n/1
  Product/1 -> b_w_r/n/1

== system CubeSat_Archiv/Simscape Plant/FeedFwd ==
  OMEGA : Inport
  omega_w : Inport  Port=2
  Demux : Demux
  G_s : Gain  Gain=G_s  Multiplication=Matrix(u*K)
  I_RW : Gain  Gain=I_rw  Multiplication=Matrix(u*K)
  Mux : Mux
  Product : Product  Multiplication=Matrix(*)
  Product1 : Product  Multiplication=Matrix(*)
  RW 1 : Subsystem
  RW 2 : Subsystem
  RW 3 : Subsystem
  RW 4 : Subsystem
  Vector Cross Product : MATLAB Function  TreatAsAtomicUnit=on
  Vector Cross Product1 : MATLAB Function  TreatAsAtomicUnit=on
  Out Bus Element : Outport  PortName=FeedFwd  Element=1
  Out Bus Element1 : Outport  PortName=FeedFwd  Element=2
  wires:
  Demux/2 -> RW 2/2(omega_w_1)
  RW 2/1(h_w_1) -> Mux/2
  Demux/4 -> RW 4/2(omega_w_1)
  OMEGA/1 -> Product/2, RW 4/1(OMEGA), RW 3/1(OMEGA), RW 2/1(OMEGA), RW 1/1(OMEGA), Vector Cross Product1/1(u), Vector Cross Product/1(u)
  Mux/1 -> Product1/2
  RW 4/1(h_w_1) -> Mux/4
  Demux/1 -> RW 1/2(omega_w_1)
  RW 1/1(h_w_1) -> Mux/1
  RW 3/1(h_w_1) -> Mux/3
  Demux/3 -> RW 3/2(omega_w_1)
  Vector Cross Product/1(u_tilde) -> I_RW/1
  Product/1 -> Out Bus Element/1
  I_RW/1 -> Product/1
  G_s/1 -> Product1/1
  Vector Cross Product1/1(u_tilde) -> G_s/1
  omega_w/1 -> Demux/1
  Product1/1 -> Out Bus Element1/1

== system CubeSat_Archiv/Simscape Plant/Kinematics1 ==
  OMEGA : Inport
  Constant : Constant  Value=0
  Gain : Gain  Gain=0.5
  Integrator : Integrator  InitialCondition=quat_0
  Quaternion Multiplication : aerolibutil/Quaternion Multiplication
  Quaternion Normalize : sharedutil/Quaternion Normalize  aMode=aMode
      settings: SourceProductName=Aerospace Blockset  SourceProductBaseCode=AE
  Vector Concatenate : Concatenate
  q : Outport
  wires:
  Quaternion Multiplication/1 -> Integrator/1
  OMEGA/1 -> Vector Concatenate/2
  Integrator/1 -> Quaternion Normalize/1, Gain/1
  Gain/1 -> Quaternion Multiplication/1
  Vector Concatenate/1 -> Quaternion Multiplication/2
  Constant/1 -> Vector Concatenate/1
  Quaternion Normalize/1 -> q/1
